simulink model "Lab8"  (R2017a)
settings: Solver=VariableStepAuto  StartTime=0.0  StopTime=30  RelTol=1e-5
undefined symbols (not defined in the file): K, T_1, T_2
settings Model: Creator=User  LastModifiedBy=User

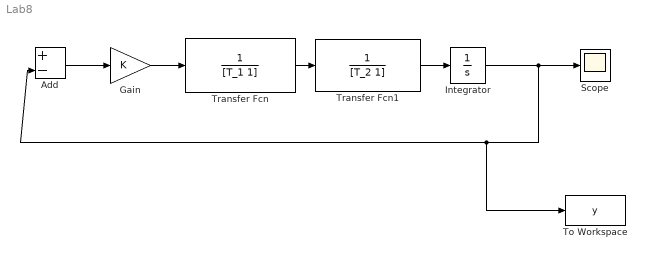
== system Lab8 ==
  Add : Sum  Inputs=+-
  Gain : Gain  Gain=K
  Integrator : Integrator  InitialCondition=1
  Scope : Scope
  To Workspace : ToWorkspace  VariableName=y  SampleTime=-1
  Transfer Fcn : TransferFcn  Denominator=[T_1 1]
  Transfer Fcn1 : TransferFcn  Denominator=[T_2 1]
  wires:
  Transfer Fcn/1 -> Transfer Fcn1/1
  Transfer Fcn1/1 -> Integrator/1
  Gain/1 -> Transfer Fcn/1
  Add/1 -> Gain/1
  Integrator/1 -> Scope/1, To Workspace/1, Add/2
